simulink model "zadacha_16"  (Simulink 7.1)
settings: Solver=ode45  StartTime=0.0  StopTime=250  RelTol=1e-3
settings Model: Creator=Slavi  LastModifiedBy=Slavi

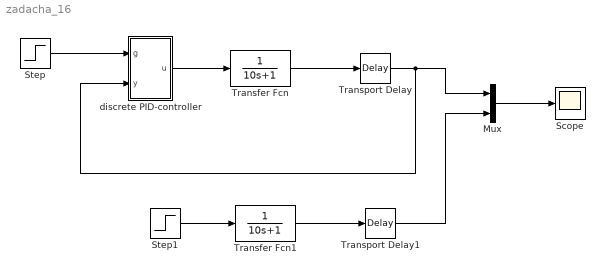
== system zadacha_16 ==
  Mux : Mux  Inputs=2
  Scope : Scope
  Step : Step
  Step1 : Step
  Transfer Fcn : TransferFcn  Denominator=[10 1]
  Transfer Fcn1 : TransferFcn  Denominator=[10 1]
  Transport Delay : TransportDelay  DelayTime=2
  Transport Delay1 : TransportDelay  DelayTime=2
  discrete PID-controller : Subsystem  mask(PID_REG){P=1, I=25, D=1, T=1}
      mask prompts: P "P="; I "I="; D "D="; T "T="
      mask help: PID discrete controller
      mask init:
      | q2=P*D/T;
      | q0=P+q2;
      | q1=-P+P*T/I-2*q2;
      mask Help: enter P,I,D,T
  wires:
  discrete PID-controller/1(u) -> Transfer Fcn/1
  Mux/1 -> Scope/1
  Transfer Fcn/1 -> Transport Delay/1
  Transport Delay/1 -> Mux/1, discrete PID-controller/2(y)
  Transfer Fcn1/1 -> Transport Delay1/1
  Transport Delay1/1 -> Mux/2
  Step/1 -> discrete PID-controller/1(g)
  Step1/1 -> Transfer Fcn1/1

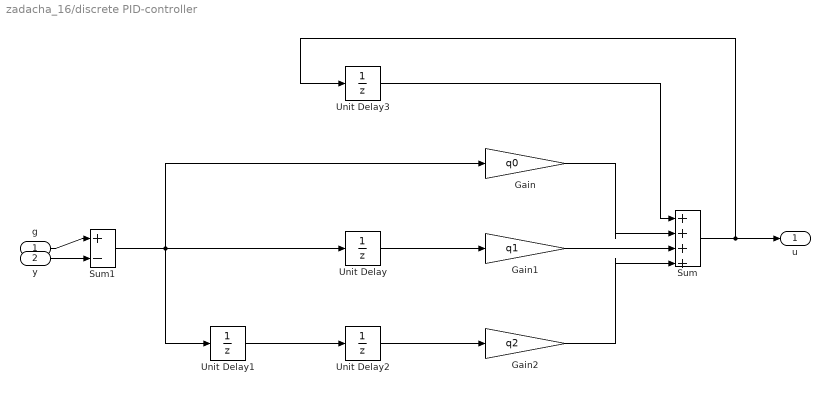
== system zadacha_16/discrete PID-controller ==
  g : Inport
  y : Inport  Port=2
  Gain : Gain  Gain=q0  ParameterDataType=sfix(16)  ParameterScaling=2^0  OutDataType=sfix(16)  OutScaling=2^0
  Gain1 : Gain  Gain=q1  ParameterDataType=sfix(16)  ParameterScaling=2^0  OutDataType=sfix(16)  OutScaling=2^0
  Gain2 : Gain  Gain=q2  ParameterDataType=sfix(16)  ParameterScaling=2^0  OutDataType=sfix(16)  OutScaling=2^0
  Sum : Sum  Inputs=|++++  OutDataType=sfix(16)  OutScaling=2^0
  Sum1 : Sum  Inputs=|+-  OutDataType=sfix(16)  OutScaling=2^0
  Unit Delay{,1..3} (4 alike) : UnitDelay
  u : Outport  OutDataType=sfix(16)  OutScaling=2^0
  wires:
  Unit Delay/1 -> Gain1/1
  Unit Delay2/1 -> Gain2/1
  Unit Delay1/1 -> Unit Delay2/1
  Gain/1 -> Sum/2
  Gain1/1 -> Sum/3
  Gain2/1 -> Sum/4
  Sum/1 -> Unit Delay3/1, u/1
  Unit Delay3/1 -> Sum/1
  Sum1/1 -> Unit Delay/1, Gain/1, Unit Delay1/1
  g/1 -> Sum1/1
  y/1 -> Sum1/2
